simulink model "Lecture24_Sim"  (R2021b)
settings: Solver=FixedStepAuto  StartTime=0.0  StopTime=20  FixedStep=0.01  RelTol=1e-3
InitFcn:
  | Lecture24_Highwire;
undefined symbols (not defined in the file): A, B, C, K, KLQR, L, LLQE, x0, xhat0
settings Model: Creator=vcichella  LastModifiedBy=vcichella
settings SolverCC: AlgebraicLoopSolver=TrustRegion
settings DebuggingCC: SFMachineParentedDataDiag=warning

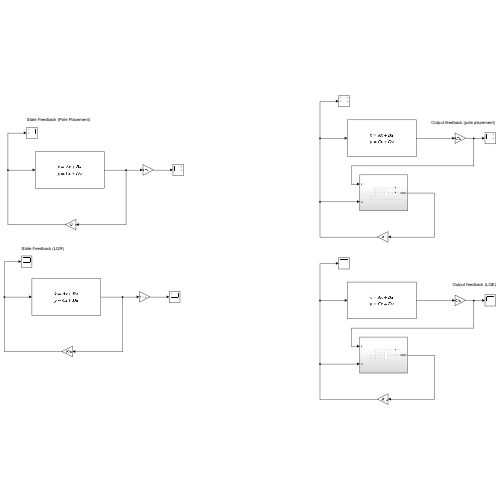
[thumbnail: Simulink's stored preview of the top-level diagram]
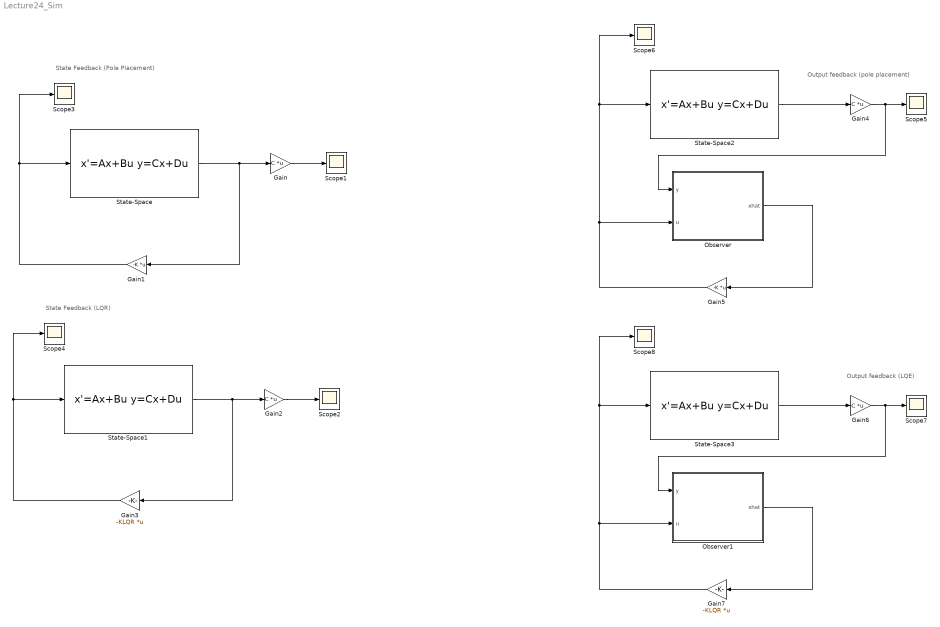
== system Lecture24_Sim ==
  note: Output feedback (LQE)
  note: Output feedback (pole placement)
  note: State Feedback (LQR)
  note: State Feedback (Pole Placement)
  Gain{,2,4,6} (4 alike) : Gain  Gain=C  Multiplication=Matrix(K*u)
  Gain1 : Gain  Gain=-K  Multiplication=Matrix(K*u)
  Gain3 : Gain  Gain=-KLQR  Multiplication=Matrix(K*u)
  Gain5 : Gain  Gain=-K  Multiplication=Matrix(K*u)
  Gain7 : Gain  Gain=-KLQR  Multiplication=Matrix(K*u)
  Observer : Subsystem
  Observer1 : Subsystem
  Scope{1..8} (8 alike) : Scope
  State-Space{,1..3} (4 alike) : StateSpace  A=A  B=B  C=eye(4)  D=zeros(4,1)  InitialCondition=x0
  wires:
  State-Space/1 -> Gain1/1, Gain/1
  Gain/1 -> Scope1/1
  Gain1/1 -> Scope3/1, State-Space/1
  Gain3/1 -> Scope4/1, State-Space1/1
  Gain2/1 -> Scope2/1
  State-Space1/1 -> Gain2/1, Gain3/1
  Gain5/1 -> Observer/2(u), State-Space2/1, Scope6/1
  Gain4/1 -> Observer/1(y), Scope5/1
  State-Space2/1 -> Gain4/1
  Observer/1(xhat) -> Gain5/1
  Observer1/1(xhat) -> Gain7/1
  State-Space3/1 -> Gain6/1
  Gain6/1 -> Scope7/1, Observer1/1(y)
  Gain7/1 -> Scope8/1, State-Space3/1, Observer1/2(u)

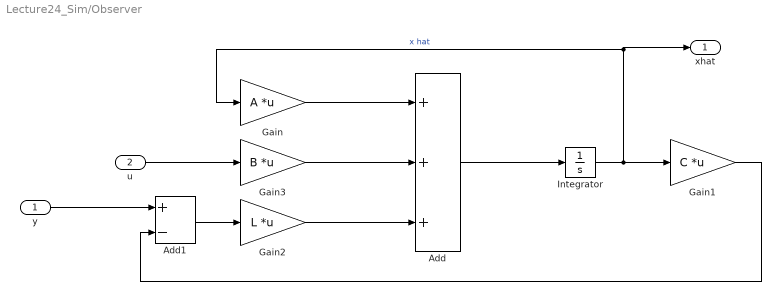
== system Lecture24_Sim/Observer ==
  y : Inport
  u : Inport  Port=2
  Add : Sum  Inputs=+++
  Add1 : Sum  Inputs=+-
  Gain : Gain  Gain=A  Multiplication=Matrix(K*u)
  Gain1 : Gain  Gain=C  Multiplication=Matrix(K*u)
  Gain2 : Gain  Gain=L  Multiplication=Matrix(K*u)
  Gain3 : Gain  Gain=B  Multiplication=Matrix(K*u)
  Integrator : Integrator  InitialCondition=xhat0
  xhat : Outport
  wires:
  Integrator/1 -> xhat/1, Gain/1, Gain1/1  "x hat"
  Add/1 -> Integrator/1
  Gain/1 -> Add/1
  Gain1/1 -> Add1/2
  Add1/1 -> Gain2/1
  y/1 -> Add1/1
  Gain2/1 -> Add/3
  u/1 -> Gain3/1
  Gain3/1 -> Add/2

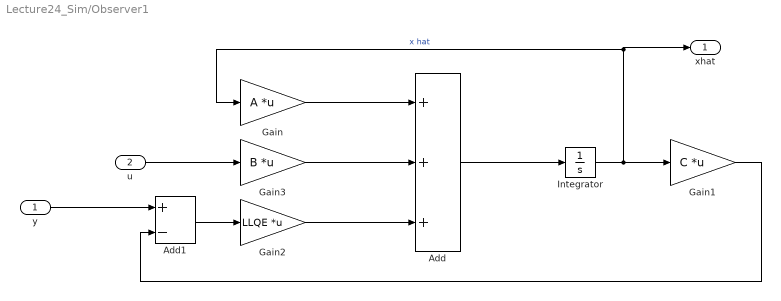
== system Lecture24_Sim/Observer1 ==
  y : Inport
  u : Inport  Port=2
  Add : Sum  Inputs=+++
  Add1 : Sum  Inputs=+-
  Gain : Gain  Gain=A  Multiplication=Matrix(K*u)
  Gain1 : Gain  Gain=C  Multiplication=Matrix(K*u)
  Gain2 : Gain  Gain=LLQE  Multiplication=Matrix(K*u)
  Gain3 : Gain  Gain=B  Multiplication=Matrix(K*u)
  Integrator : Integrator  InitialCondition=xhat0
  xhat : Outport
  wires:
  Gain3/1 -> Add/2
  u/1 -> Gain3/1
  Gain2/1 -> Add/3
  y/1 -> Add1/1
  Add1/1 -> Gain2/1
  Gain1/1 -> Add1/2
  Gain/1 -> Add/1
  Add/1 -> Integrator/1
  Integrator/1 -> Gain1/1, Gain/1, xhat/1  "x hat"
